simulink model "linear_inverted_pendulum"  (R2025a)
settings: Solver=FixedStepAuto  StartTime=0.0  StopTime=10.0  RelTol=1e-3
undefined symbols (not defined in the file): A, B, x_0, x_op
settings Model: Creator=amoralesma  LastModifiedBy=amoralesma

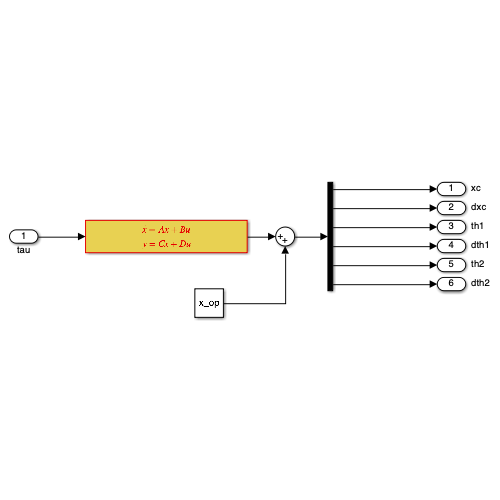
[thumbnail: Simulink's stored preview of the top-level diagram]
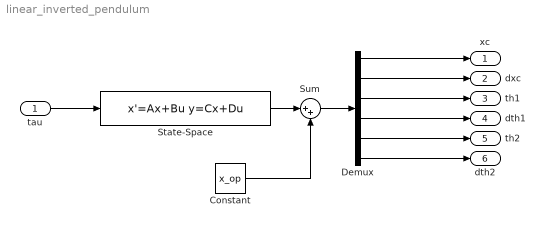
== system linear_inverted_pendulum ==
  tau : Inport
  Constant : Constant  Value=x_op
  Demux : Demux  Outputs=6
  State-Space : StateSpace  A=A  B=B  C=eye(6)  D=zeros(6, 1)  InitialCondition=x_0 - x_op
  Sum : Sum  Inputs=|++
  xc : Outport
  dxc : Outport  Port=2
  th1 : Outport  Port=3
  dth1 : Outport  Port=4
  th2 : Outport  Port=5
  dth2 : Outport  Port=6
  wires:
  Demux/2 -> dxc/1
  tau/1 -> State-Space/1
  Constant/1 -> Sum/2
  Demux/1 -> xc/1
  State-Space/1 -> Sum/1
  Demux/5 -> th2/1
  Demux/3 -> th1/1
  Demux/4 -> dth1/1
  Sum/1 -> Demux/1
  Demux/6 -> dth2/1
